simulink model "SolarCellModelShading"  (R2023a)
settings: Solver=VariableStepAuto  StartTime=0.0  StopTime=3  RelTol=1e-3
libraries: spsPVArrayLib x12, spsControlledVoltageSourceLib x1, spsCurrentMeasurementLib x1, spsDiodeLib x1, simulink x1, spsVoltageMeasurementLib x1, sps_lib x1
settings Model: Creator=hp  LastModifiedBy=ask
settings SolverCC: AlgebraicLoopSolver=TrustRegion
settings DataIOCC: ReturnWorkspaceOutputs=off
settings DebuggingCC: UnconnectedInputMsg=warning  UnconnectedOutputMsg=warning  UnconnectedLineMsg=warning  ArithmeticOperatorsInVariantConditions=warning
settings ModelReferenceCC: EnableRefExpFcnMdlSchedulingChecks=on
settings SFSimCC: SimUseLocalCustomCode=off  CustomCodeUndefinedFunction=UseInterfaceOnly
settings RTWCC: RTWUseLocalCustomCode=off
settings CodeAppCC: StateflowObjectComments=on
settings SimscapeCC: SimscapeNormalizeSystem=off

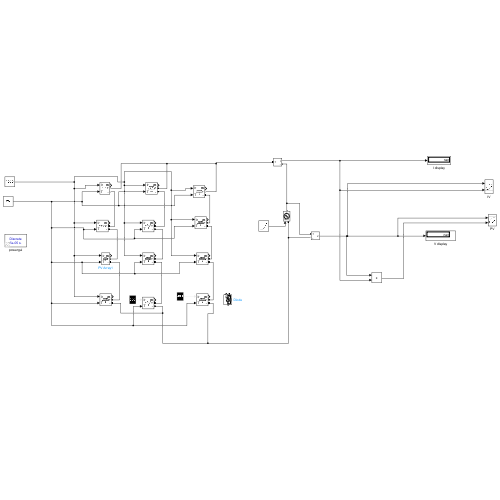
[thumbnail: Simulink's stored preview of the top-level diagram]
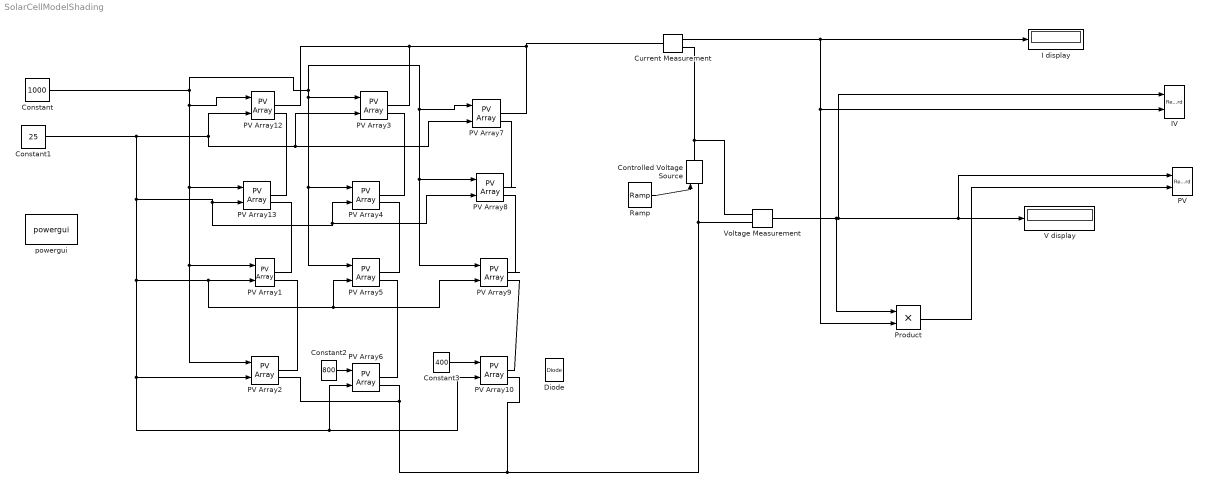
== system SolarCellModelShading ==
  Constant : Constant  Value=1000
  Constant1 : Constant  Value=25
  Constant2 : Constant  Value=800
  Constant3 : Constant  Value=400
  Controlled Voltage Source : spsControlledVoltageSourceLib/Controlled Voltage Source  Initialize=on  Source_Type=AC  Amplitude=0  Phase=0  Frequency=0  Measurements=None
  Current Measurement : spsCurrentMeasurementLib/Current Measurement  PhasorSimulation=off  OutputType=Complex  PSBequivalent=0
  Diode : spsDiodeLib/Diode  Ron=0.001  Lon=0  Vf=0.8  IC=0  UseSnubber=off  Rs=500  Cs=250e-9  Measurements=on
  I display : Display
  IV : Record  FileSettingsInternal="{\"entries\":[{\"content\":{\"excelSettings\":{\"content\":{},\"type\":\"Streamout.ExcelSettings\"}},\"type\":\"Streamout.FileSettingStorage\",\"uuid\":\"b8201c09-556e-40f2-b499-5385ed36e242\"}],\"packageUris\":[\"http://schema.mathworks.com/mf0/streamout_blocks/R2020a\"],\"version\":\"1.0\"}"  Layout=[1 1]  SignalsInternal="{\"entries\":[{\"content\":{\"signals\":[{\"content\":{\"blockPath\":[\"Shading/IV\"],\"dimensions\":[1],\"domain\":\"Shading/IV\",\"lineColor\":\"#a2142f\",\"plots\":[1],\"port\":1,\"sid\":[\"\"],\"signalID\":153,\"signalName\":\"Voltage Measurement\"},\"type\":\"RecordBlkView.Signal\",\"uuid\":\"45a29ef5-5293-4033-8d7a-232e5841ae2c\"},{\"content\":{\"blockPath\":[\"Shading/IV\"],\"dimensions\":[1],\"domain\":\"Shading/IV\",\"lineColor\":\"#139fff\",\"plots\":[1],\"port\":2,\"sid\":[\"\"],\"signalID\":157,\"signalName\":\"Current Measurement\"},\"type\":\"RecordBlkView.Signal\",\"uuid\":\"5103f835-5b35-410d-9cb6-2d7f43410f14\"}]},\"type\":\"RecordBlkView.InputSignals\",\"uuid\":\"4247cf7d-409f-4229-9695-d4d8b892ce40\"}],\"packageUris\":[\"http://schema.mathworks.com/mf0/streamout_blocks/R2020a\"],\"version\":\"1.0\"}"  VisualizationBindings="{\"xyplotplugin\":{\"info\":[{\"series\":[{\"bindingParametersList\":[{\"parameter\":\"X-Axis\",\"signalID\":153,\"signalName\":\"Voltage Measurement\"},{\"parameter\":\"Y-Axis\",\"signalID\":157,\"signalName\":\"Current Measurement\"}],\"seriesID\":54271}],\"subplotID\":1}]}}"  CompatibilityTag=XY  st=-1
  PV : Record  FileSettingsInternal="{\"entries\":[{\"content\":{\"excelSettings\":{\"content\":{},\"type\":\"Streamout.ExcelSettings\"}},\"type\":\"Streamout.FileSettingStorage\",\"uuid\":\"57b184b8-c8f9-4a4c-ba11-6740da2591bd\"}],\"packageUris\":[\"http://schema.mathworks.com/mf0/streamout_blocks/R2020a\"],\"version\":\"1.0\"}"  Layout=[1 1]  SignalsInternal="{\"entries\":[{\"content\":{\"signals\":[{\"content\":{\"blockPath\":[\"Shading/PV\"],\"dimensions\":[1],\"domain\":\"Shading/PV\",\"lineColor\":\"#a2142f\",\"plots\":[1],\"port\":1,\"sid\":[\"\"],\"signalID\":161,\"signalName\":\"Voltage Measurement\"},\"type\":\"RecordBlkView.Signal\",\"uuid\":\"5d101edc-88bd-4c16-969e-1a3dae33f3cf\"},{\"content\":{\"blockPath\":[\"Shading/PV\"],\"dimensions\":[1],\"domain\":\"Shading/PV\",\"lineColor\":\"#139fff\",\"plots\":[1],\"port\":2,\"sid\":[\"\"],\"signalID\":165,\"signalName\":\"Product\"},\"type\":\"RecordBlkView.Signal\",\"uuid\":\"65841d88-9aa4-4d69-81f0-ba7036430a53\"}]},\"type\":\"RecordBlkView.InputSignals\",\"uuid\":\"2dfd4f3c-a151-484b-97cf-65c69ec1212c\"}],\"packageUris\":[\"http://schema.mathworks.com/mf0/streamout_blocks/R2020a\"],\"version\":\"1.0\"}"  VisualizationBindings="{\"xyplotplugin\":{\"info\":[{\"series\":[{\"bindingParametersList\":[{\"parameter\":\"X-Axis\",\"signalID\":161,\"signalName\":\"Voltage Measurement\"},{\"parameter\":\"Y-Axis\",\"signalID\":165,\"signalName\":\"Product\"}],\"seriesID\":53125}],\"subplotID\":1}]}}"  CompatibilityTag=XY  st=-1
  PV Array{1..10,12..13} (12 alike) : spsPVArrayLib/PV Array  Npar=1  Nser=1  PlotType=array @ 1000 W/m2 & specified temperatures  S_vec="[ 1000  500  100 ]"  Temp_C_vec="[ 45 25  ]"  ModuleName=User-defined  PlotWhenSelected=off  Pm=213.15  Ncell=60  Voc=36.3  Isc=7.84  Vm=29  Im=7.35  beta_Voc_pc=-0.36099  alpha_Isc_pc=0.102  beta_Voc=-0.13104  alpha_Isc=0.0079968  IL=7.8654  I0=2.9273e-10  nI=0.98119  Rsh=313.0553  Rs=0.39381  RobustModel=off  RobustCellTemperature=313.3991  BAL=on  Tc=1e-6  Tfilter=5e-5
  Product : Product
  Ramp : simulink/Sources/Ramp  slope=145.2  start=0  InitialOutput=0
  V display : Display
  Voltage Measurement : spsVoltageMeasurementLib/Voltage Measurement  PhasorSimulation=off  OutputType=Complex  PSBequivalent=0
  powergui : sps_lib/powergui  Priority=1  SimulationMode=Discrete  SampleTime=50e-6  frequency=60  Iterations=50  frequencyindice=0  Pbase=100e6  ErrMax=1e-4  UnitsV=kV  UnitsW=MW  buscounter=0  FunctionMessages=off  echomessages=off  EnableUseOfTLC=off  CurrentSourceSwitches=off  DisableSnubberDevices=off  DisableRonSwitches=off  DisableVfSwitches=off  DisplayEquations=off  AutomaticDiscreteSolvers=off  SolverType=Tustin/Backward Euler (TBE)  Interpol=off  ExternalGateDelay=off  methode=off  Ts=10  x0status=blocks  SPID=off  SwTol=0  HookPort=off  NonlinearTolerance=1e-4  nMaxIteration=100  ContinueOnMaxIteration=off  RestoreLinks=warning  ResistiveCurrentMeasurement=off  Frange=[0:2:500]  Ylog=off  Xlog=on  ShowGrid=off  save=off  variable=ZData  structure=0  ZoomFFT=off  StartTime=0.0  cycles=1  DisplayStyle=1  fundamental=60  FreqAxis=off  MaxFrequency=1000  frequencyindicesteady=1  RmsSteady=1  display=off
  wires:
  Constant/1 -> PV Array12/1, PV Array13/1, PV Array2/1, PV Array1/1, PV Array5/1, PV Array4/1, PV Array3/1, PV Array7/1, PV Array9/1, PV Array8/1
  Constant1/1 -> PV Array12/2, PV Array7/2, PV Array3/2, PV Array13/2, PV Array8/2, PV Array4/2, PV Array9/2, PV Array5/2, PV Array1/2, PV Array10/2, PV Array6/2, PV Array2/2
  Ramp/1 -> Controlled Voltage Source/1
  Current Measurement/1 -> Product/2, IV/2, I display/1
  Product/1 -> PV/2
  Voltage Measurement/1 -> PV/1, V display/1, IV/1, Product/1
  Constant3/1 -> PV Array10/1
  Constant2/1 -> PV Array6/1
  connections:
  PV Array7/RConn1 -- Current Measurement/LConn1 -- PV Array3/RConn1 -- PV Array12/RConn1
  Controlled Voltage Source/RConn1 -- Current Measurement/RConn1 -- Voltage Measurement/LConn1
  Controlled Voltage Source/LConn1 -- PV Array10/RConn2 -- PV Array6/RConn2 -- PV Array2/RConn2 -- Voltage Measurement/LConn2
  PV Array1/RConn2 -- PV Array2/RConn1
  PV Array13/RConn2 -- PV Array1/RConn1
  PV Array9/RConn1 -- PV Array8/RConn2
  PV Array4/RConn1 -- PV Array3/RConn2
  PV Array13/RConn1 -- PV Array12/RConn2
  PV Array5/RConn2 -- PV Array6/RConn1
  PV Array8/RConn1 -- PV Array7/RConn2
  PV Array5/RConn1 -- PV Array4/RConn2
  PV Array9/RConn2 -- PV Array10/RConn1
